simulink model "ex6"  (R2019b)
settings: Solver=FixedStepAuto  StartTime=0.0  StopTime=inf  FixedStep=FIXED_STEP_SIZE  RelTol=1e-3
model workspace (MAT data in the model file):
  SL_ROS_VariableLengthArrays_MaxSizes.CommonInfo.ArrayTruncateAction = 'EmitWarning'
  SL_ROS_VariableLengthArrays_MaxSizes.MsgTypeMap = containers.Map
  SL_ROS_VariableLengthArrays_MaxSizes.MsgTypeMap.serialization.keys = {'mav_msgs/Actuators'}
  SL_ROS_VariableLengthArrays_MaxSizes.MsgTypeMap.serialization.values{1}(1).PropertyName = 'Angles'
  SL_ROS_VariableLengthArrays_MaxSizes.MsgTypeMap.serialization.values{1}(1).DataType = 'double'
  SL_ROS_VariableLengthArrays_MaxSizes.MsgTypeMap.serialization.values{1}(1).MaxLength = 128
  SL_ROS_VariableLengthArrays_MaxSizes.MsgTypeMap.serialization.values{1}(2).PropertyName = 'AngularVelocities'
  SL_ROS_VariableLengthArrays_MaxSizes.MsgTypeMap.serialization.values{1}(2).DataType = 'double'
  SL_ROS_VariableLengthArrays_MaxSizes.MsgTypeMap.serialization.values{1}(2).MaxLength = 4
  SL_ROS_VariableLengthArrays_MaxSizes.MsgTypeMap.serialization.values{1}(3).PropertyName = 'Normalized'
  SL_ROS_VariableLengthArrays_MaxSizes.MsgTypeMap.serialization.values{1}(3).DataType = 'double'
  SL_ROS_VariableLengthArrays_MaxSizes.MsgTypeMap.serialization.values{1}(3).MaxLength = 128
  SL_ROS_VariableLengthArrays_MaxSizes.MsgTypeMap.serialization.uniformity = 0
  SL_ROS_VariableLengthArrays_MaxSizes.MsgTypeMap.serialization.keyType = 'char'
  SL_ROS_VariableLengthArrays_MaxSizes.MsgTypeMap.serialization.valueType = 'any'
values from neighbouring files (symbols this model uses):
  B = 1.3678e-7    (= 1.3678e-07)    [motor_velocity_interface_main.m]
  FIXED_STEP_SIZE = 0.01    [motor_velocity_interface_main.m]
  GRAVITY = 9.81    [motor_velocity_interface_main.m]
  IXX = 0.007    [motor_velocity_interface_main.m]
  IYY = 0.007    [motor_velocity_interface_main.m]
  IZZ = 0.012    [motor_velocity_interface_main.m]
  K = 8.54858e-6    (= 8.54858e-06)    [motor_velocity_interface_main.m]
  L = 0.17    [motor_velocity_interface_main.m]
  MASS = 0.716    [motor_velocity_interface_main.m]
  MAX_ROTOR_VEL = 838    [motor_velocity_interface_main.m]
undefined symbols (not defined in the file or in its folder): AngularVelocities, AngularVelocities_SL_Info, Header
libraries: robotlib x5, simulink x4, robotgazebolib x1
settings Model: Creator=ananda  LastModifiedBy=ubuntu
settings OptimizationCC: EnhancedBackFolding=on  PassReuseOutputArgsAs=Individual arguments  ZeroExternalMemoryAtStartup=off  ZeroInternalMemoryAtStartup=off  MaxStackSize=64  OptimizeBlockOrder=speed  DifferentSizesBufferReuse=on  OptimizationCustomize=off  EfficientTunableParamExpr=on
settings DebuggingCC: ParameterTunabilityLossMsg=error
settings HardwareCC: ProdBitPerPointer=32  ProdBitPerSizeT=32  ProdBitPerPtrDiffT=32  ProdLargestAtomicFloat=None  ProdIntDivRoundTo=Undefined  ProdEndianess=Unspecified  ProdWordSize=32  ProdHWDeviceType=Generic->Unspecified (assume 32-bit Generic)  UseEmbeddedCoderFeatures=off
settings SFSimCC: MATLABDynamicMemAlloc=off
settings RTWCC: SystemTargetFile=ert.tlc  HardwareBoard=Robot Operating System (ROS)  TLCOptions="-aInlineSetEventsForThisBaseRateFcn=TLC_FALSE -aSuppressMultiTaskScheduler=TLC_FALSE  -aRateBasedStepFcn=0"  TemplateMakefile=ert_default_tmf  GenerateReport=on  Toolchain=Catkin  IncludeHyperlinkInReport=on  LaunchReport=on  TargetLang=C++  GenerateTraceInfo=on  GenerateTraceReport=on  GenerateTraceReportSl=on  GenerateTraceReportSf=on  GenerateTraceReportEml=on
settings CodeAppCC: ForceParamTrailComments=on  IgnoreCustomStorageClasses=off  OperatorAnnotations=on  SimulinkDataObjDesc=on  SFDataObjDesc=on  InsertBlockDesc=on
settings ERTTargetCC: SupportNonInlinedSFcns=on

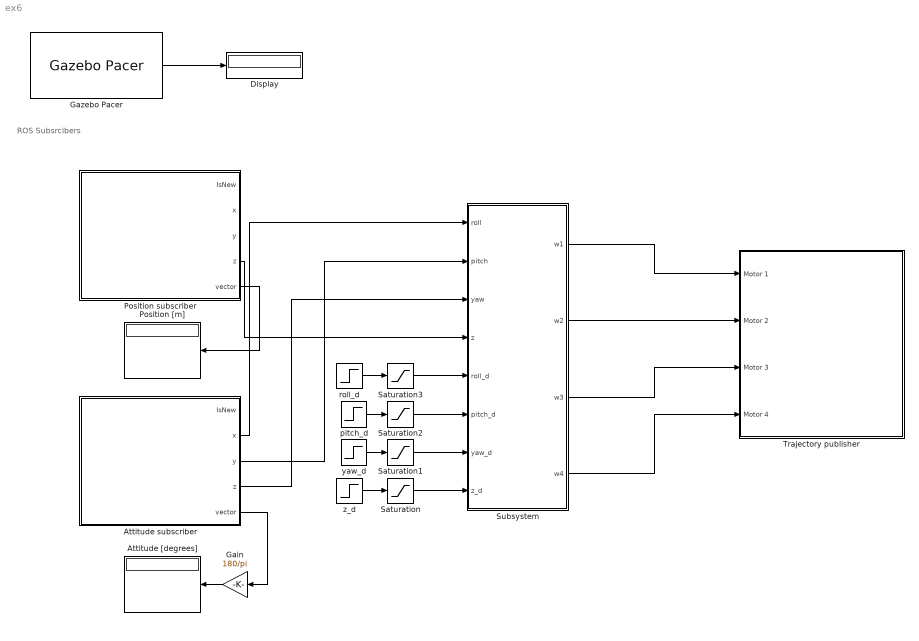
== system ex6 ==
  note: ROS Subsrcibers
  Attitude [degrees] : Display
  Attitude subscriber : Subsystem
  Display : Display
  Gain : Gain  Gain=180/pi
  Gazebo Pacer : robotgazebolib/Gazebo Pacer  ResetBehavior=Reset Gazebo simulation time  SampleTime=FIXED_STEP_SIZE
      settings: SourceProductName=Robotics System Toolbox  SourceProductBaseCode=RO
  Position [m] : Display
  Position subscriber : Subsystem
  Saturation : Saturate  UpperLimit=inf  LowerLimit=0.06
  Saturation1 : Saturate  UpperLimit=pi  LowerLimit=-pi
  Saturation2 : Saturate  UpperLimit=pi  LowerLimit=-pi
  Saturation3 : Saturate  UpperLimit=pi  LowerLimit=-pi
  Subsystem : Subsystem
  Trajectory publisher : Subsystem
  pitch_d : Step  Time=0.1  After=0  SampleTime=0
  roll_d : Step  After=pi/18  SampleTime=0
  yaw_d : Step  Time=0.1  After=0  SampleTime=0
  z_d : Step  Time=0.1  SampleTime=0
  wires:
  Position subscriber/5(vector) -> Position [m]/1
  Attitude subscriber/5(vector) -> Gain/1
  Gain/1 -> Attitude [degrees]/1
  Gazebo Pacer/1 -> Display/1
  Subsystem/1(w1) -> Trajectory publisher/1(Motor 1)
  Subsystem/2(w2) -> Trajectory publisher/2(Motor 2)
  Subsystem/3(w3) -> Trajectory publisher/3(Motor 3)
  Subsystem/4(w4) -> Trajectory publisher/4(Motor 4)
  Attitude subscriber/2(x) -> Subsystem/1(roll)
  Attitude subscriber/3(y) -> Subsystem/2(pitch)
  Attitude subscriber/4(z) -> Subsystem/3(yaw)
  Position subscriber/4(z) -> Subsystem/4(z)
  z_d/1 -> Saturation/1
  Saturation/1 -> Subsystem/8(z_d)
  roll_d/1 -> Saturation3/1
  Saturation3/1 -> Subsystem/5(roll_d)
  Saturation2/1 -> Subsystem/6(pitch_d)
  Saturation1/1 -> Subsystem/7(yaw_d)
  yaw_d/1 -> Saturation1/1
  pitch_d/1 -> Saturation2/1

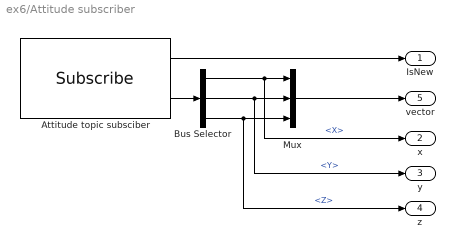
== system ex6/Attitude subscriber ==
  Attitude topic subsciber : robotlib/Subscribe  topicSource=Specify your own  topic=/hummingbird/orientation_rpy  messageType=geometry_msgs/Vector3  sampleTime=ATTI_SUB_DT  messageQueueLength=1
      settings: SourceProductName=ROS Toolbox
  Bus Selector : BusSelector  OutputSignals=X,Y,Z
  Mux : Mux  Inputs=3
  IsNew : Outport
  x : Outport  Port=2
  y : Outport  Port=3
  z : Outport  Port=4
  vector : Outport  Port=5
  wires:
  Bus Selector/3 -> z/1, Mux/3  "<Z>"
  Bus Selector/2 -> y/1, Mux/2  "<Y>"
  Bus Selector/1 -> x/1, Mux/1  "<X>"
  Attitude topic subsciber/2 -> Bus Selector/1
  Attitude topic subsciber/1 -> IsNew/1
  Mux/1 -> vector/1

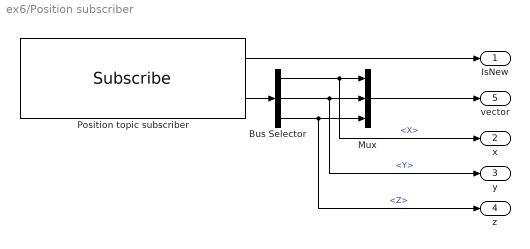
== system ex6/Position subscriber ==
  Bus Selector : BusSelector  OutputSignals=Point.X,Point.Y,Point.Z
  Mux : Mux  Inputs=3
  Position topic subscriber : robotlib/Subscribe  topicSource=Specify your own  topic=/hummingbird/odometry_sensor1/position  messageType=geometry_msgs/PointStamped  sampleTime=POS_SUB_DT  messageQueueLength=1
      settings: SourceProductName=ROS Toolbox
  IsNew : Outport
  x : Outport  Port=2
  y : Outport  Port=3
  z : Outport  Port=4
  vector : Outport  Port=5
  wires:
  Bus Selector/3 -> z/1, Mux/3  "<Z>"
  Bus Selector/2 -> y/1, Mux/2  "<Y>"
  Mux/1 -> vector/1
  Bus Selector/1 -> x/1, Mux/1  "<X>"
  Position topic subscriber/2 -> Bus Selector/1
  Position topic subscriber/1 -> IsNew/1

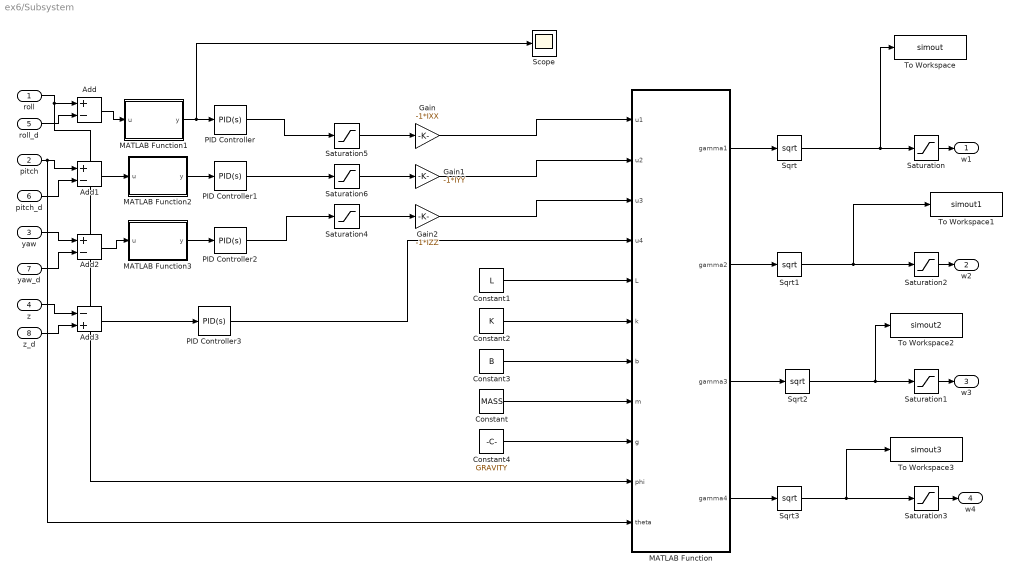
== system ex6/Subsystem ==
  roll : Inport
  pitch : Inport  Port=2
  yaw : Inport  Port=3
  z : Inport  Port=4
  roll_d : Inport  Port=5
  pitch_d : Inport  Port=6
  yaw_d : Inport  Port=7
  z_d : Inport  Port=8
  Add : Sum  Inputs=+-
  Add1 : Sum  Inputs=+-
  Add2 : Sum  Inputs=+-
  Add3 : Sum  Inputs=-+
  Constant : Constant  Value=MASS
  Constant1 : Constant  Value=L
  Constant2 : Constant  Value=K
  Constant3 : Constant  Value=B
  Constant4 : Constant  Value=GRAVITY
  Gain : Gain  Gain=-1*IXX
  Gain1 : Gain  Gain=-1*IYY
  Gain2 : Gain  Gain=-1*IZZ
  MATLAB Function : MATLAB Function  TreatAsAtomicUnit=on
  MATLAB Function1 : MATLAB Function  TreatAsAtomicUnit=on
  MATLAB Function2 : MATLAB Function  TreatAsAtomicUnit=on
  MATLAB Function3 : MATLAB Function  TreatAsAtomicUnit=on
  PID Controller : simulink/Continuous/PID Controller  Controller=PID  Form=Parallel  TimeDomain=Continuous-time  SampleTime=-1  IntegratorMethod=Forward Euler  FilterMethod=Forward Euler  ControllerParametersSource=internal  P=3  I=0.1  D=1.5  UseFilter=on  N=100  TunerSelectOption=Transfer Function Based (PID Tuner App)  InitialConditionSource=internal  InitialConditionForIntegrator=0  InitialConditionForFilter=0  DifferentiatorICPrevScaledInput=0  ExternalReset=none  TrackingMode=off  Kt=1  LimitOutput=off  UpperSaturationLimit=inf  LowerSaturationLimit=-inf  LinearizeAsGain=on  AntiWindupMode=none  Kb=1  POutMin=[]  POutMax=[]  IOutMin=[]  IOutMax=[]  DOutMin=[]  DOutMax=[]  NOutMin=[]  NOutMax=[]  SumOutMin=[]  SumOutMax=[]  SaturationOutMin=[]  SaturationOutMax=[]  PParamMin=[]  PParamMax=[]  IParamMin=[]  IParamMax=[]  DParamMin=[]  DParamMax=[]  NParamMin=[]  NParamMax=[]  KbParamMin=[]  KbParamMax=[]  KtParamMin=[]  KtParamMax=[]  KbOutMin=[]  KbOutMax=[]  KtOutMin=[]  KtOutMax=[]  IntegratorOutMin=[]  IntegratorOutMax=[]  FilterOutMin=[]  FilterOutMax=[]  SumI1OutMin=[]  SumI1OutMax=[]  SumI2OutMin=[]  SumI2OutMax=[]  SumI3OutMin=[]  SumI3OutMax=[]  SumI4OutMin=[]  SumI4OutMax=[]  SumDOutMin=[]  SumDOutMax=[]  DifferentiatorOutMin=[]  DifferentiatorOutMax=[]  FilterDiffOutCoefMin=[]  FilterDiffOutCoefMax=[]  ReciprocalOutMin=[]  ReciprocalOutMax=[]  SumDenOutMin=[]  SumDenOutMax=[]  SumNumOutMin=[]  SumNumOutMax=[]  DivideOutMin=[]  DivideOutMax=[]  IntegratorContinuousStateAttributes=''  IntegratorStateMustResolveToSignalObject=off  IntegratorRTWStateStorageClass=Auto  FilterContinuousStateAttributes=''  FilterStateMustResolveToSignalObject=off  FilterRTWStateStorageClass=Auto  ParallelPVariant=InternalParameters  IdealPVariant=Disabled  IVariant=InternalParameters  DVariant=InternalParameters  IntegratorVariant=Continuous  SatVariant=Disabled  AWVariant=Passthrough  PCopyVariant=Disabled  TRVariant=Disabled  FdbkBlocksVariant=Forward  IdealPFdbkVariant=Disabled  SatFdbkVariant=Disabled  DerivativeFilterVariant=ContFilter  NVariant=InternalParameters  NCopyVariant=Disabled  FilterICVariant=InternalICsFilter  IntegratorICVariant=InternalICs  ExternalResetVariant=Disabled  TRSumVariant=Passthrough  SumFdbkVariant=Disabled  SumVariant=Sum_PID
  PID Controller1 : simulink/Continuous/PID Controller  Controller=PID  Form=Parallel  TimeDomain=Continuous-time  SampleTime=-1  IntegratorMethod=Forward Euler  FilterMethod=Forward Euler  ControllerParametersSource=internal  P=3  I=0.2  D=3  UseFilter=on  N=100  TunerSelectOption=Transfer Function Based (PID Tuner App)  InitialConditionSource=internal  InitialConditionForIntegrator=0  InitialConditionForFilter=0  DifferentiatorICPrevScaledInput=0  ExternalReset=none  TrackingMode=off  Kt=1  LimitOutput=off  UpperSaturationLimit=inf  LowerSaturationLimit=-inf  LinearizeAsGain=on  AntiWindupMode=none  Kb=1  POutMin=[]  POutMax=[]  IOutMin=[]  IOutMax=[]  DOutMin=[]  DOutMax=[]  NOutMin=[]  NOutMax=[]  SumOutMin=[]  SumOutMax=[]  SaturationOutMin=[]  SaturationOutMax=[]  PParamMin=[]  PParamMax=[]  IParamMin=[]  IParamMax=[]  DParamMin=[]  DParamMax=[]  NParamMin=[]  NParamMax=[]  KbParamMin=[]  KbParamMax=[]  KtParamMin=[]  KtParamMax=[]  KbOutMin=[]  KbOutMax=[]  KtOutMin=[]  KtOutMax=[]  IntegratorOutMin=[]  IntegratorOutMax=[]  FilterOutMin=[]  FilterOutMax=[]  SumI1OutMin=[]  SumI1OutMax=[]  SumI2OutMin=[]  SumI2OutMax=[]  SumI3OutMin=[]  SumI3OutMax=[]  SumI4OutMin=[]  SumI4OutMax=[]  SumDOutMin=[]  SumDOutMax=[]  DifferentiatorOutMin=[]  DifferentiatorOutMax=[]  FilterDiffOutCoefMin=[]  FilterDiffOutCoefMax=[]  ReciprocalOutMin=[]  ReciprocalOutMax=[]  SumDenOutMin=[]  SumDenOutMax=[]  SumNumOutMin=[]  SumNumOutMax=[]  DivideOutMin=[]  DivideOutMax=[]  IntegratorContinuousStateAttributes=''  IntegratorStateMustResolveToSignalObject=off  IntegratorRTWStateStorageClass=Auto  FilterContinuousStateAttributes=''  FilterStateMustResolveToSignalObject=off  FilterRTWStateStorageClass=Auto  ParallelPVariant=InternalParameters  IdealPVariant=Disabled  IVariant=InternalParameters  DVariant=InternalParameters  IntegratorVariant=Continuous  SatVariant=Disabled  AWVariant=Passthrough  PCopyVariant=Disabled  TRVariant=Disabled  FdbkBlocksVariant=Forward  IdealPFdbkVariant=Disabled  SatFdbkVariant=Disabled  DerivativeFilterVariant=ContFilter  NVariant=InternalParameters  NCopyVariant=Disabled  FilterICVariant=InternalICsFilter  IntegratorICVariant=InternalICs  ExternalResetVariant=Disabled  TRSumVariant=Passthrough  SumFdbkVariant=Disabled  SumVariant=Sum_PID
  PID Controller2 : simulink/Continuous/PID Controller  Controller=PID  Form=Parallel  TimeDomain=Continuous-time  SampleTime=-1  IntegratorMethod=Forward Euler  FilterMethod=Forward Euler  ControllerParametersSource=internal  P=5  I=0.2  D=3  UseFilter=on  N=100  TunerSelectOption=Transfer Function Based (PID Tuner App)  InitialConditionSource=internal  InitialConditionForIntegrator=0  InitialConditionForFilter=0  DifferentiatorICPrevScaledInput=0  ExternalReset=none  TrackingMode=off  Kt=1  LimitOutput=off  UpperSaturationLimit=inf  LowerSaturationLimit=-inf  LinearizeAsGain=on  AntiWindupMode=none  Kb=1  POutMin=[]  POutMax=[]  IOutMin=[]  IOutMax=[]  DOutMin=[]  DOutMax=[]  NOutMin=[]  NOutMax=[]  SumOutMin=[]  SumOutMax=[]  SaturationOutMin=[]  SaturationOutMax=[]  PParamMin=[]  PParamMax=[]  IParamMin=[]  IParamMax=[]  DParamMin=[]  DParamMax=[]  NParamMin=[]  NParamMax=[]  KbParamMin=[]  KbParamMax=[]  KtParamMin=[]  KtParamMax=[]  KbOutMin=[]  KbOutMax=[]  KtOutMin=[]  KtOutMax=[]  IntegratorOutMin=[]  IntegratorOutMax=[]  FilterOutMin=[]  FilterOutMax=[]  SumI1OutMin=[]  SumI1OutMax=[]  SumI2OutMin=[]  SumI2OutMax=[]  SumI3OutMin=[]  SumI3OutMax=[]  SumI4OutMin=[]  SumI4OutMax=[]  SumDOutMin=[]  SumDOutMax=[]  DifferentiatorOutMin=[]  DifferentiatorOutMax=[]  FilterDiffOutCoefMin=[]  FilterDiffOutCoefMax=[]  ReciprocalOutMin=[]  ReciprocalOutMax=[]  SumDenOutMin=[]  SumDenOutMax=[]  SumNumOutMin=[]  SumNumOutMax=[]  DivideOutMin=[]  DivideOutMax=[]  IntegratorContinuousStateAttributes=''  IntegratorStateMustResolveToSignalObject=off  IntegratorRTWStateStorageClass=Auto  FilterContinuousStateAttributes=''  FilterStateMustResolveToSignalObject=off  FilterRTWStateStorageClass=Auto  ParallelPVariant=InternalParameters  IdealPVariant=Disabled  IVariant=InternalParameters  DVariant=InternalParameters  IntegratorVariant=Continuous  SatVariant=Disabled  AWVariant=Passthrough  PCopyVariant=Disabled  TRVariant=Disabled  FdbkBlocksVariant=Forward  IdealPFdbkVariant=Disabled  SatFdbkVariant=Disabled  DerivativeFilterVariant=ContFilter  NVariant=InternalParameters  NCopyVariant=Disabled  FilterICVariant=InternalICsFilter  IntegratorICVariant=InternalICs  ExternalResetVariant=Disabled  TRSumVariant=Passthrough  SumFdbkVariant=Disabled  SumVariant=Sum_PID
  PID Controller3 : simulink/Continuous/PID Controller  Controller=PID  Form=Parallel  TimeDomain=Continuous-time  SampleTime=-1  IntegratorMethod=Forward Euler  FilterMethod=Forward Euler  ControllerParametersSource=internal  P=5  I=0.3  D=3  UseFilter=on  N=100  TunerSelectOption=Transfer Function Based (PID Tuner App)  InitialConditionSource=internal  InitialConditionForIntegrator=0  InitialConditionForFilter=0  DifferentiatorICPrevScaledInput=0  ExternalReset=none  TrackingMode=off  Kt=1  LimitOutput=off  UpperSaturationLimit=inf  LowerSaturationLimit=-inf  LinearizeAsGain=on  AntiWindupMode=none  Kb=1  POutMin=[]  POutMax=[]  IOutMin=[]  IOutMax=[]  DOutMin=[]  DOutMax=[]  NOutMin=[]  NOutMax=[]  SumOutMin=[]  SumOutMax=[]  SaturationOutMin=[]  SaturationOutMax=[]  PParamMin=[]  PParamMax=[]  IParamMin=[]  IParamMax=[]  DParamMin=[]  DParamMax=[]  NParamMin=[]  NParamMax=[]  KbParamMin=[]  KbParamMax=[]  KtParamMin=[]  KtParamMax=[]  KbOutMin=[]  KbOutMax=[]  KtOutMin=[]  KtOutMax=[]  IntegratorOutMin=[]  IntegratorOutMax=[]  FilterOutMin=[]  FilterOutMax=[]  SumI1OutMin=[]  SumI1OutMax=[]  SumI2OutMin=[]  SumI2OutMax=[]  SumI3OutMin=[]  SumI3OutMax=[]  SumI4OutMin=[]  SumI4OutMax=[]  SumDOutMin=[]  SumDOutMax=[]  DifferentiatorOutMin=[]  DifferentiatorOutMax=[]  FilterDiffOutCoefMin=[]  FilterDiffOutCoefMax=[]  ReciprocalOutMin=[]  ReciprocalOutMax=[]  SumDenOutMin=[]  SumDenOutMax=[]  SumNumOutMin=[]  SumNumOutMax=[]  DivideOutMin=[]  DivideOutMax=[]  IntegratorContinuousStateAttributes=''  IntegratorStateMustResolveToSignalObject=off  IntegratorRTWStateStorageClass=Auto  FilterContinuousStateAttributes=''  FilterStateMustResolveToSignalObject=off  FilterRTWStateStorageClass=Auto  ParallelPVariant=InternalParameters  IdealPVariant=Disabled  IVariant=InternalParameters  DVariant=InternalParameters  IntegratorVariant=Continuous  SatVariant=Disabled  AWVariant=Passthrough  PCopyVariant=Disabled  TRVariant=Disabled  FdbkBlocksVariant=Forward  IdealPFdbkVariant=Disabled  SatFdbkVariant=Disabled  DerivativeFilterVariant=ContFilter  NVariant=InternalParameters  NCopyVariant=Disabled  FilterICVariant=InternalICsFilter  IntegratorICVariant=InternalICs  ExternalResetVariant=Disabled  TRSumVariant=Passthrough  SumFdbkVariant=Disabled  SumVariant=Sum_PID
  Saturation{,1..3} (4 alike) : Saturate  UpperLimit=MAX_ROTOR_VEL  LowerLimit=0
  Saturation4 : Saturate  UpperLimit=4  LowerLimit=-4
  Saturation5 : Saturate  UpperLimit=0.4  LowerLimit=-0.4
  Saturation6 : Saturate  UpperLimit=0.4  LowerLimit=-0.4
  Scope : Scope
  Sqrt{,1..3} (4 alike) : Sqrt  SaturateOnIntegerOverflow=on
  To Workspace : ToWorkspace  VariableName=simout  SaveFormat=Timeseries  SampleTime=-1
  To Workspace1 : ToWorkspace  VariableName=simout1  SaveFormat=Timeseries  SampleTime=-1
  To Workspace2 : ToWorkspace  VariableName=simout2  SaveFormat=Timeseries  SampleTime=-1
  To Workspace3 : ToWorkspace  VariableName=simout3  SaveFormat=Timeseries  SampleTime=-1
  w1 : Outport
  w2 : Outport  Port=2
  w3 : Outport  Port=3
  w4 : Outport  Port=4
  wires:
  roll/1 -> MATLAB Function/10(phi), Add/1
  roll_d/1 -> Add/2
  pitch/1 -> MATLAB Function/11(theta), Add1/1
  pitch_d/1 -> Add1/2
  yaw/1 -> Add2/1
  yaw_d/1 -> Add2/2
  z/1 -> Add3/1
  z_d/1 -> Add3/2
  Add3/1 -> PID Controller3/1
  Gain/1 -> MATLAB Function/1(u1)
  Gain1/1 -> MATLAB Function/2(u2)
  Gain2/1 -> MATLAB Function/3(u3)
  Constant3/1 -> MATLAB Function/7(b)
  Constant1/1 -> MATLAB Function/5(L)
  MATLAB Function/1(gamma1) -> Sqrt/1
  MATLAB Function/2(gamma2) -> Sqrt1/1
  MATLAB Function/3(gamma3) -> Sqrt2/1
  MATLAB Function/4(gamma4) -> Sqrt3/1
  Saturation/1 -> w1/1
  Saturation1/1 -> w3/1
  Saturation2/1 -> w2/1
  Saturation3/1 -> w4/1
  Constant2/1 -> MATLAB Function/6(k)
  PID Controller3/1 -> MATLAB Function/4(u4)
  Constant/1 -> MATLAB Function/8(m)
  Constant4/1 -> MATLAB Function/9(g)
  PID Controller2/1 -> Saturation4/1
  MATLAB Function1/1(y) -> Scope/1, PID Controller/1
  Add/1 -> MATLAB Function1/1(u)
  MATLAB Function2/1(y) -> PID Controller1/1
  Add1/1 -> MATLAB Function2/1(u)
  Add2/1 -> MATLAB Function3/1(u)
  MATLAB Function3/1(y) -> PID Controller2/1
  Saturation4/1 -> Gain2/1
  PID Controller/1 -> Saturation5/1
  PID Controller1/1 -> Saturation6/1
  Saturation5/1 -> Gain/1
  Saturation6/1 -> Gain1/1
  Sqrt1/1 -> To Workspace1/1, Saturation2/1
  Sqrt/1 -> To Workspace/1, Saturation/1
  Sqrt2/1 -> To Workspace2/1, Saturation1/1
  Sqrt3/1 -> To Workspace3/1, Saturation3/1

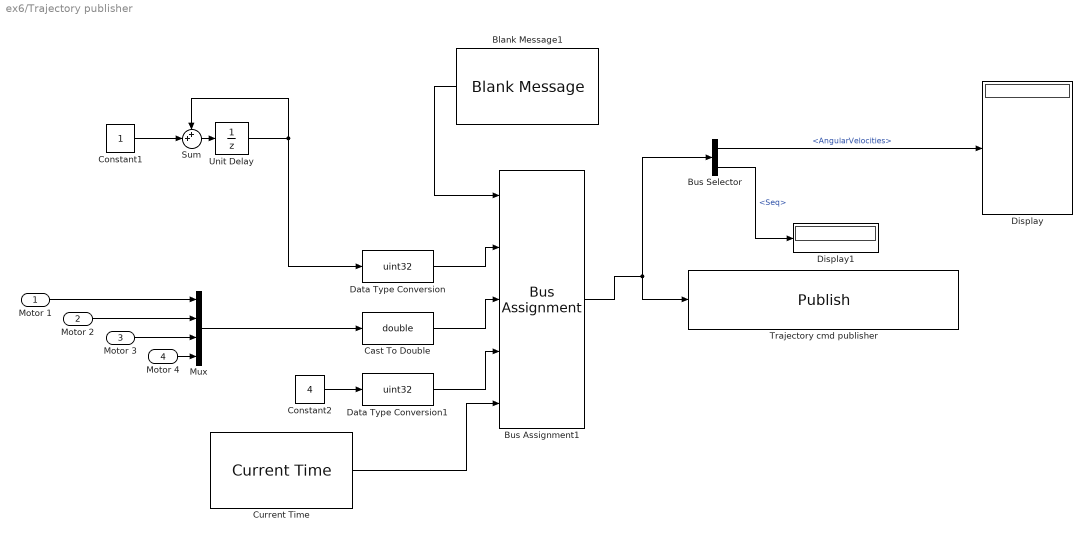
== system ex6/Trajectory publisher ==
  Motor 1 : Inport
  Motor 2 : Inport  Port=2
  Motor 3 : Inport  Port=3
  Motor 4 : Inport  Port=4
  Blank Message1 : robotlib/Blank Message  messageClass=Message  entityType=mav_msgs/Actuators  messageType=mav_msgs/Actuators  SampleTime=inf
      settings: SourceProductName=ROS Toolbox
  Bus Assignment1 : BusAssignment  AssignedSignals=Header.Seq,AngularVelocities,AngularVelocities_SL_Info.CurrentLength,Header.Stamp
  Bus Selector : BusSelector  OutputSignals=AngularVelocities,Header.Seq
  Cast To Double : DataTypeConversion  OutDataTypeStr=double
  Constant1 : Constant
  Constant2 : Constant  Value=4
  Current Time : robotlib/Current Time  OutputFormat=bus  SampleTime=FIXED_STEP_SIZE  ModelName=ex6
      settings: SourceProductName=ROS Toolbox  SourceProductBaseCode=RR
  Data Type Conversion : DataTypeConversion  OutDataTypeStr=uint32
  Data Type Conversion1 : DataTypeConversion  OutDataTypeStr=uint32
  Display : Display
  Display1 : Display
  Mux : Mux
  Sum : Sum  Inputs=++|
  Trajectory cmd publisher : robotlib/Publish  topicSource=Specify your own  topic=/hummingbird/command/motor_speed  messageType=mav_msgs/Actuators  messageQueueLength=1
      settings: SourceProductName=ROS Toolbox
  Unit Delay : UnitDelay  SampleTime=FIXED_STEP_SIZE  HasFrameUpgradeWarning=on
  wires:
  Bus Assignment1/1 -> Trajectory cmd publisher/1, Bus Selector/1
  Blank Message1/1 -> Bus Assignment1/1
  Data Type Conversion/1 -> Bus Assignment1/2
  Mux/1 -> Cast To Double/1
  Cast To Double/1 -> Bus Assignment1/3
  Bus Selector/1 -> Display/1  "<AngularVelocities>"
  Bus Selector/2 -> Display1/1  "<Seq>"
  Constant2/1 -> Data Type Conversion1/1
  Data Type Conversion1/1 -> Bus Assignment1/4
  Motor 1/1 -> Mux/1
  Motor 2/1 -> Mux/2
  Motor 3/1 -> Mux/3
  Motor 4/1 -> Mux/4
  Current Time/1 -> Bus Assignment1/5
  Sum/1 -> Unit Delay/1
  Unit Delay/1 -> Data Type Conversion/1, Sum/1
  Constant1/1 -> Sum/2

== matlab function ex6/Subsystem/MATLAB Function1 ==
  data: u input; y output
function y = fcn(u)
if abs(u)>pi
   y = u - 2*u/abs(u)*pi;
else
    y = u;
end
end

== matlab function ex6/Subsystem/MATLAB Function ==
  data: gamma1 output double; gamma2 output double; gamma3 output double; gamma4 output double; u1 input; u2 input; u3 input; u4 input; L input; k input; b input; m input; g input; phi input; theta input
function [gamma1, gamma2, gamma3, gamma4]= fcn(u1, u2, u3, u4, L, k, b, m, g, phi, theta)
A = (m*g+m*u4)/(k*cos(phi)*cos(theta));
% M = [0, L*k, 0, -L*k;
%     -L*k, 0, L*k, 0;
%     b, -b, b, -b;
%     1,1,1,1];
ux = u1/(L*k);
uy = u2/(L*k);
uz = u3/b;
gamma3 = (A+2*uy+uz)/4;
gamma4 = (A-2*ux-uz)/4;
gamma1 = gamma3-uy;
gamma2 = ux+gamma4;
gamma1 = max([gamma1,0]);
gamma2 = max([gamma2,0]);
gamma3 = max([gamma3,0]);
gamma4 = max([gamma4,0]);
end

== matlab function ex6/Subsystem/MATLAB Function2 ==
  data: u input; y output
function y = fcn(u)
if abs(u)>pi
   y = u - 2*u/abs(u)*pi;
else
    y = u;
end
end

== matlab function ex6/Subsystem/MATLAB Function3 ==
  data: u input; y output
function y = fcn(u)
if abs(u)>pi
   y = u - 2*u/abs(u)*pi;
else
    y = u;
end
end
